simulink model "rossler_attractor"  (R2024b)
settings: Solver=ode45  StartTime=0.0  StopTime=100  RelTol=1e-3
settings Model: Creator=Botló  LastModifiedBy=Botló

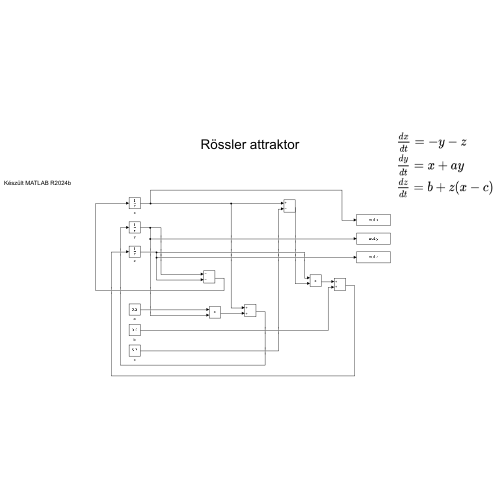
[thumbnail: Simulink's stored preview of the top-level diagram]
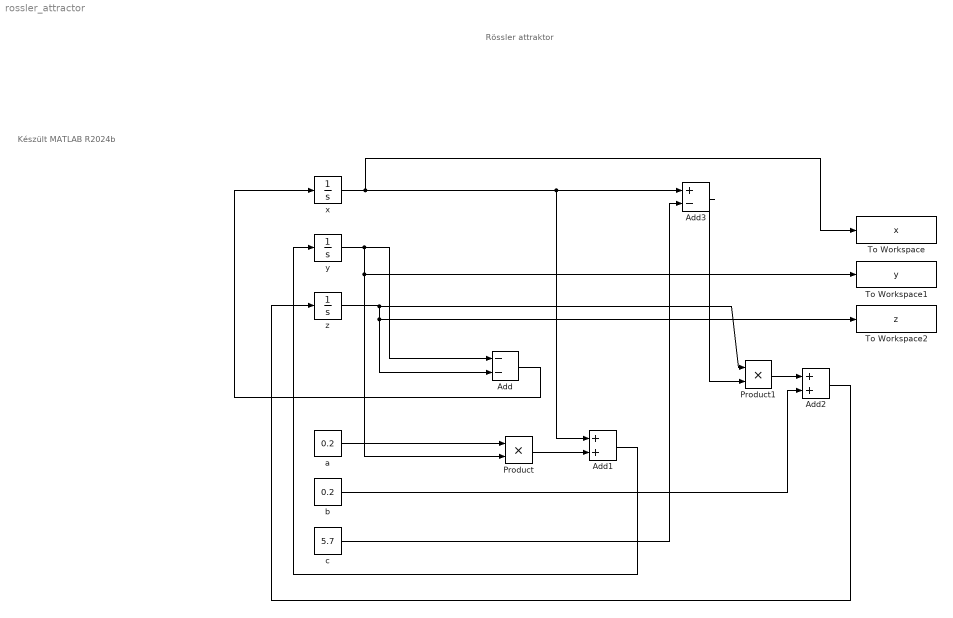
== system rossler_attractor ==
  note: Készült MATLAB R2024b
  note: Rössler attraktor
  Add : Sum  Inputs=--
  Add1 : Sum
  Add2 : Sum
  Add3 : Sum  Inputs=+-
  Product : Product
  Product1 : Product
  To Workspace : ToWorkspace  VariableName=x  SampleTime=-1
      settings: Save2DSignal=2-D array (concatenate along first dimension)
  To Workspace1 : ToWorkspace  VariableName=y  SampleTime=-1
      settings: Save2DSignal=2-D array (concatenate along first dimension)
  To Workspace2 : ToWorkspace  VariableName=z  SampleTime=-1
      settings: Save2DSignal=2-D array (concatenate along first dimension)
  a : Constant  Value=0.2
  b : Constant  Value=0.2
  c : Constant  Value=5.7
  x : Integrator  InitialCondition=1
  y : Integrator
  z : Integrator
  wires:
  y/1 -> To Workspace1/1, Product/2, Add/1
  z/1 -> To Workspace2/1, Add/2, Product1/1
  Add/1 -> x/1
  Product/1 -> Add1/2
  a/1 -> Product/1
  Add1/1 -> y/1
  x/1 -> To Workspace/1, Add3/1, Add1/1
  c/1 -> Add3/2
  Add3/1 -> Product1/2
  Product1/1 -> Add2/1
  b/1 -> Add2/2
  Add2/1 -> z/1
